simulink model "gyak10_matlabgyak2_sim"  (R2015a)
settings: Solver=ode45  StartTime=0.0  StopTime=100.0  RelTol=1e-3
libraries: commnoisgen2 x3
settings Model: Creator=ppolcz  LastModifiedBy=ppolcz

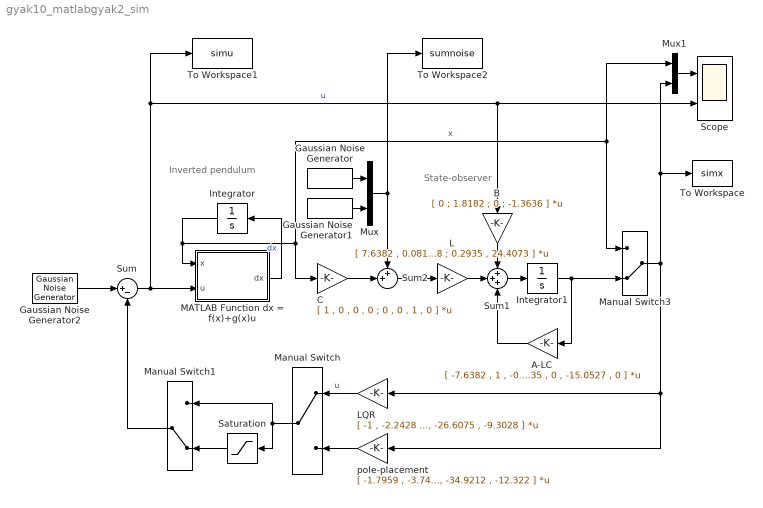
== system gyak10_matlabgyak2_sim ==
  note: State-observer
  note: Inverted pendulum
  A-LC : Gain  Gain=[ -7.6382 , 1 , -0.0811 , 0 ; -14.5773 , -0 , -0.3123 , 0 ; -0.0761 , 0 , -7.7618 , 1 ; -0.2935 , 0 , -15.0527 , 0 ]  Multiplication=Matrix(K*u)
  B : Gain  Gain=[ 0 ; 1.8182 ; 0 ; -1.3636 ]  Multiplication=Matrix(K*u)
  C : Gain  Gain=[ 1 , 0 , 0 , 0 ; 0 , 0 , 1 , 0 ]  Multiplication=Matrix(K*u)
  Gaussian Noise Generator : commnoisgen2/Gaussian Noise Generator  m=0  d=0.001  s=41  Ts=1  frameBased=off  sampPerFrame=1  orient=off  outDataType=double
  Gaussian Noise Generator1 : commnoisgen2/Gaussian Noise Generator  m=0  d=0.001  s=41  Ts=1  frameBased=off  sampPerFrame=1  orient=off  outDataType=double
  Gaussian Noise Generator2 : commnoisgen2/Gaussian Noise Generator  m=0  d=0.001  s=41  Ts=1  frameBased=off  sampPerFrame=1  orient=off  outDataType=double
  Integrator : Integrator  InitialCondition=[0;0;0.1;0]
  Integrator1 : Integrator  InitialCondition=[0;0;0.8;0]
  L : Gain  Gain=[ 7.6382 , 0.0811 ; 14.5773 , -2.3605 ; 0.0761 , 7.7618 ; 0.2935 , 24.4073 ]  Multiplication=Matrix(K*u)
  LQR : Gain  Gain=[ -1 , -2.2428 , -26.6075 , -9.3028 ]  Multiplication=Matrix(K*u)
  MATLAB Function dx = f(x)+g(x)u : MATLAB Function  TreatAsAtomicUnit=on
  Manual Switch : ManualSwitch
  Manual Switch1 : ManualSwitch  CurrentSetting=0
  Manual Switch3 : ManualSwitch  CurrentSetting=0
  Mux : Mux  Inputs=2
  Mux1 : Mux  Inputs=2
  Saturation : Saturate  UpperLimit=10  LowerLimit=-10
  Scope : Scope  NumInputPorts=2
      settings: YMin=-5~-5  YMax=5~5
  Sum : Sum  Inputs=|+-
  Sum1 : Sum  Inputs=+++
  Sum2 : Sum  Inputs=++|
  To Workspace : ToWorkspace  VariableName=simx  SaveFormat=Timeseries  SampleTime=-1
  To Workspace1 : ToWorkspace  VariableName=simu  SaveFormat=Timeseries  SampleTime=-1
  To Workspace2 : ToWorkspace  VariableName=sumnoise  SaveFormat=Timeseries  SampleTime=-1
  pole-placement : Gain  Gain=[ -1.7959 , -3.7415 , -34.9212 , -12.322 ]  Multiplication=Matrix(K*u)
  wires:
  MATLAB Function dx = f(x)+g(x)u/1(dx) -> Integrator/1  "dx"
  Sum/1 -> B/1, Scope/2, To Workspace1/1, MATLAB Function dx = f(x)+g(x)u/2(u)  "u"
  LQR/1 -> Manual Switch/1  "u"
  pole-placement/1 -> Manual Switch/2
  Saturation/1 -> Manual Switch1/2
  Manual Switch/1 -> Saturation/1, Manual Switch1/1
  Manual Switch1/1 -> Sum/2
  Integrator/1 -> MATLAB Function dx = f(x)+g(x)u/1(x), Manual Switch3/1, Mux1/1, C/1  "x"
  Manual Switch3/1 -> Mux1/2, To Workspace/1, pole-placement/1, LQR/1
  Sum1/1 -> Integrator1/1
  L/1 -> Sum1/2
  Integrator1/1 -> A-LC/1, Manual Switch3/2
  A-LC/1 -> Sum1/3
  B/1 -> Sum1/1
  Sum2/1 -> L/1
  C/1 -> Sum2/2
  Gaussian Noise Generator/1 -> Mux/1
  Gaussian Noise Generator1/1 -> Mux/2
  Mux/1 -> Sum2/1, To Workspace2/1
  Mux1/1 -> Scope/1
  Gaussian Noise Generator2/1 -> Sum/1

== matlab function gyak10_matlabgyak2_sim/MATLAB Function dx = f(x)+g(x)u ==
  data: x input; u input; dx output
function dx = invpend(x,u)

% model parameters
M = 0.5;
m = 0.2;
l = 1;
g = 9.8;
b = 0;

% state variables
%r = x(1);
v = x(2);
phi = x(3);
omega = x(4);

q = 4*(M+m) - 3*m*cos(phi)^2;

f = [
    v
    (4*m*l*sin(phi)*omega^2 - 1.5*m*g*sin(2*phi) -4*b*v) / q
    omega
    3*(-m*l*sin(2*phi)*omega^2 / 2 + (M+m)*g*sin(phi) + b*cos(phi)*v) / (l*q)
    ];

g = [
    0
    4*l
    0
    -3*cos(phi)
    ] / (l*q);

dx = f + g*u;

end
